simulink model "augmentedtest"  (R2020b)
settings: Solver=VariableStepAuto  StartTime=0.0  StopTime=5  RelTol=1e-3
values from neighbouring files (symbols this model uses):
  B_f = 1189    [halfcarparameters.mat]
  K = lqr(A,B,Q_pd,rho_pd)    [accel_jerk_ctrl_testbed.m]    (also in quartersuspensionscript.m)
  K_f = 66793    [halfcarparameters.mat]
  K_tf = 201021    [halfcarparameters.mat]
  m_s = 879.35    [halfcarparameters.mat]
  m_uf = 43.76    [halfcarparameters.mat]
settings Model: Creator=anishabhangui  LastModifiedBy=anishabhangui

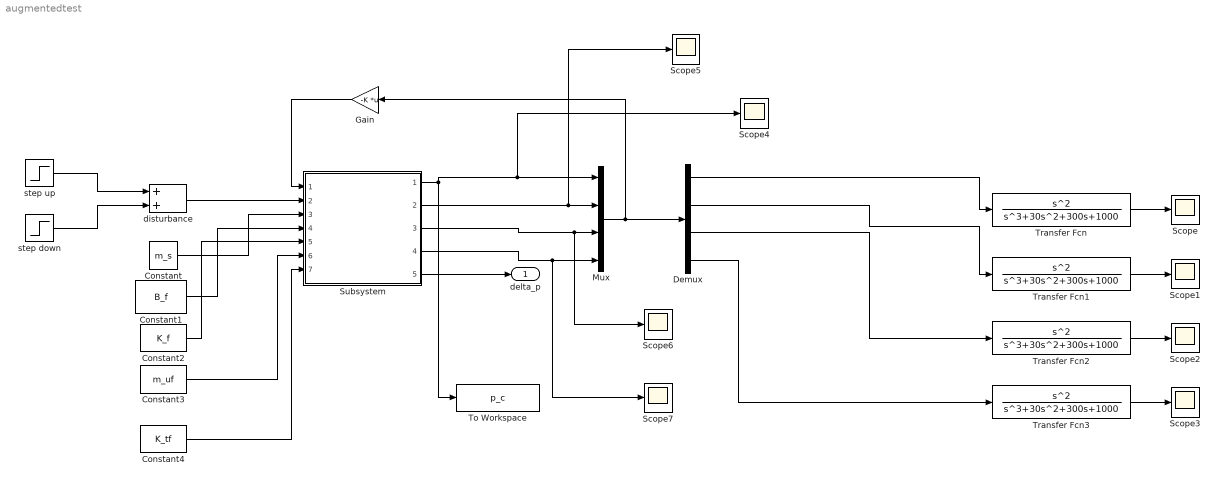
== system augmentedtest ==
  Constant : Constant  Value=m_s
  Constant1 : Constant  Value=B_f
  Constant2 : Constant  Value=K_f
  Constant3 : Constant  Value=m_uf
  Constant4 : Constant  Value=K_tf
  Demux : Demux
  Gain : Gain  Gain=-K  Multiplication=Matrix(K*u)
  Mux : Mux
  Scope{,1..7} (8 alike) : Scope
  Subsystem : Subsystem  TreatAsAtomicUnit=on  ReferencedSubsystem=quarter_car_w_tire_subsystem
  To Workspace : ToWorkspace  VariableName=p_c  SaveFormat=Timeseries  SampleTime=-1
  Transfer Fcn{,1..3} (4 alike) : TransferFcn  Numerator=[1 0 0]  Denominator=[1 30 300 1000]
  disturbance : Sum
  step down : Step  After=-1  SampleTime=0
  step up : Step  Time=0  SampleTime=0
  delta_p : Outport  VectorParamsAs1DForOutWhenUnconnected=off
  wires:
  Constant1/1 -> Subsystem/4
  step up/1 -> disturbance/1
  Constant/1 -> Subsystem/3
  disturbance/1 -> Subsystem/2
  step down/1 -> disturbance/2
  Constant3/1 -> Subsystem/6
  Constant4/1 -> Subsystem/7
  Subsystem/5 -> delta_p/1
  Constant2/1 -> Subsystem/5
  Subsystem/1 -> Scope4/1, Mux/1, To Workspace/1
  Subsystem/2 -> Scope5/1, Mux/2
  Subsystem/3 -> Scope6/1, Mux/3
  Subsystem/4 -> Scope7/1, Mux/4
  Mux/1 -> Demux/1, Gain/1
  Gain/1 -> Subsystem/1
  Demux/2 -> Transfer Fcn1/1
  Transfer Fcn2/1 -> Scope2/1
  Transfer Fcn3/1 -> Scope3/1
  Transfer Fcn1/1 -> Scope1/1
  Demux/4 -> Transfer Fcn3/1
  Demux/3 -> Transfer Fcn2/1
  Demux/1 -> Transfer Fcn/1
  Transfer Fcn/1 -> Scope/1
